simulink model "UG_Drive_System"  (R2019b)
settings: Solver=ode45  StartTime=0.0  StopTime=T_sim_d_ug  MaxStep=1e-5  RelTol=1e-3
values from neighbouring files (symbols this model uses):
  A_t = r * m * g * sin(theta)    [C2_Preliminary_Controller_Design.m]    (also in D1_Preliminary_Controller_Design.m; D2_Controller_Design.m; D3_PL_Controller_Design.m; D4_DPDZ_Controller_Design.m)
  B_t = r * C_r * m * g    [C2_Preliminary_Controller_Design.m]    (also in D1_Preliminary_Controller_Design.m = 0.0188352; D2_Controller_Design.m = 0.0188352; D3_PL_Controller_Design.m = 0.006309792; D4_DPDZ_Controller_Design.m = 0.006309792)
  C_t = r * 0.5 * rho_air * C_d * A    [C2_Preliminary_Controller_Design.m]    (also in D1_Preliminary_Controller_Design.m = 3.6e-05; D2_Controller_Design.m = 3.6e-05; D3_PL_Controller_Design.m = 3.6e-05; D4_DPDZ_Controller_Design.m = 3.6e-05)
  c_tv = r/((r.^2) * m + Jaxle)    [C2_Preliminary_Controller_Design.m]    (also in D1_Preliminary_Controller_Design.m; D2_Controller_Design.m; D3_PL_Controller_Design.m; D4_DPDZ_Controller_Design.m)
  delay_theta = 10    [D1_Preliminary_Controller_Design.m]    (also in D2_Controller_Design.m; D3_PL_Controller_Design.m; D4_DPDZ_Controller_Design.m)
  delay_v_x_ref = 1    [D1_Preliminary_Controller_Design.m]    (also in D2_Controller_Design.m; D3_PL_Controller_Design.m; D4_DPDZ_Controller_Design.m)
  eta_g_d = 1    [C2_Preliminary_Controller_Design.m]    (also in D1_Preliminary_Controller_Design.m = 0.95; D2_Controller_Design.m = 0.95; D3_PL_Controller_Design.m = 0.95; D4_DPDZ_Controller_Design.m = 0.95)
  i_a_max = 1.2    [D1_Preliminary_Controller_Design.m]    (also in D2_Controller_Design.m; D3_PL_Controller_Design.m; D4_DPDZ_Controller_Design.m)
  k_m_d =     [C2_Preliminary_Controller_Design.m]    (also in D1_Preliminary_Controller_Design.m = 0.02; D2_Controller_Design.m = 0.02; D3_PL_Controller_Design.m = 0.02; D4_DPDZ_Controller_Design.m = 0.02)
  L_a_d =     [C2_Preliminary_Controller_Design.m]    (also in D1_Preliminary_Controller_Design.m = 0.000278; D2_Controller_Design.m = 0.000278; D3_PL_Controller_Design.m = 0.000278; D4_DPDZ_Controller_Design.m = 0.000278)
  n_g_d =     [C2_Preliminary_Controller_Design.m]    (also in D1_Preliminary_Controller_Design.m = 50; D2_Controller_Design.m = 50; D3_PL_Controller_Design.m = 50; D4_DPDZ_Controller_Design.m = 50)
  pole_PL_d = exp(pole_PL_a * T_s)    [MPZ_PL.m]
  r =     [C2_Preliminary_Controller_Design.m]    (also in D1_Preliminary_Controller_Design.m = 0.06; D2_Controller_Design.m = 0.06; D3_PL_Controller_Design.m = 0.06; D4_DPDZ_Controller_Design.m = 0.06)
  R_a_d =     [C2_Preliminary_Controller_Design.m]    (also in D1_Preliminary_Controller_Design.m = 2.19; D2_Controller_Design.m = 2.19; D3_PL_Controller_Design.m = 2.19; D4_DPDZ_Controller_Design.m = 2.19)
  v_x_ref = 0.15    [D1_Preliminary_Controller_Design.m]    (also in D2_Controller_Design.m = 0.4; D3_PL_Controller_Design.m = 0.02; D4_DPDZ_Controller_Design.m = 0.02)
  zero_PL_d = exp(zero_PL_a * T_s)    [MPZ_PL.m]
undefined symbols (not defined in the file or in its folder): K_PL_d
settings Model: Creator=Conor  LastModifiedBy=Conor Healy
settings DataIOCC: SaveOutput=off  SignalLogging=off  DSMLogging=off  SaveTime=off  ReturnWorkspaceOutputs=off
settings SFSimCC: CustomCodeUndefinedFunction=UseInterfaceOnly

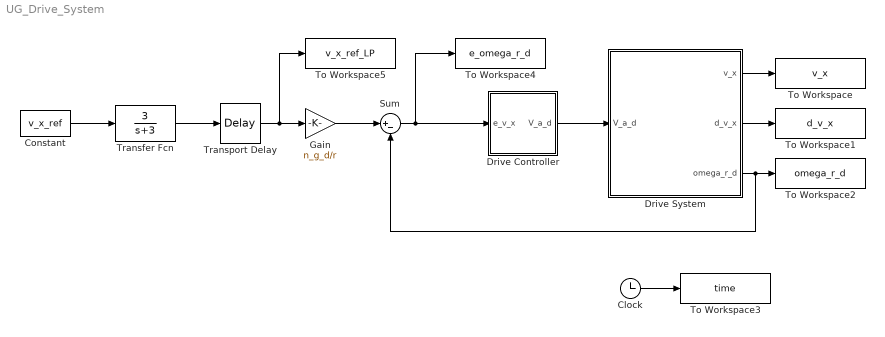
== system UG_Drive_System ==
  Clock : Clock
  Constant : Constant  Value=v_x_ref
  Drive Controller : Subsystem
  Drive System : Subsystem
  Gain : Gain  Gain=n_g_d/r
      settings: AttributesFormatString=%<Gain>
  Sum : Sum  Inputs=|+-
  To Workspace : ToWorkspace  VariableName=v_x  SampleTime=-1
  To Workspace1 : ToWorkspace  VariableName=d_v_x  SampleTime=-1
  To Workspace2 : ToWorkspace  VariableName=omega_r_d  SampleTime=-1
  To Workspace3 : ToWorkspace  VariableName=time  SampleTime=-1
  To Workspace4 : ToWorkspace  VariableName=e_omega_r_d  SampleTime=-1
  To Workspace5 : ToWorkspace  VariableName=v_x_ref_LP  SampleTime=-1
  Transfer Fcn : TransferFcn  Numerator=[3]  Denominator=[1 3]
  Transport Delay : TransportDelay  DelayTime=delay_v_x_ref  BufferSize=4096
  wires:
  Drive System/1(v_x) -> To Workspace/1
  Drive System/2(d_v_x) -> To Workspace1/1
  Drive System/3(omega_r_d) -> Sum/2, To Workspace2/1
  Gain/1 -> Sum/1
  Clock/1 -> To Workspace3/1
  Transport Delay/1 -> To Workspace5/1, Gain/1
  Sum/1 -> Drive Controller/1(e_v_x), To Workspace4/1
  Transfer Fcn/1 -> Transport Delay/1
  Constant/1 -> Transfer Fcn/1
  Drive Controller/1(V_a_d) -> Drive System/1(V_a_d)

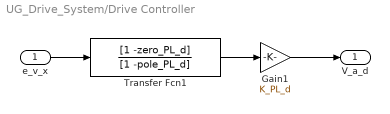
== system UG_Drive_System/Drive Controller ==
  e_v_x : Inport
  Gain1 : Gain  Gain=K_PL_d
      settings: AttributesFormatString=%<Gain>
  Transfer Fcn1 : TransferFcn  Numerator=[1 -zero_PL_d]  Denominator=[1 -pole_PL_d]
  V_a_d : Outport
  wires:
  Transfer Fcn1/1 -> Gain1/1
  Gain1/1 -> V_a_d/1
  e_v_x/1 -> Transfer Fcn1/1

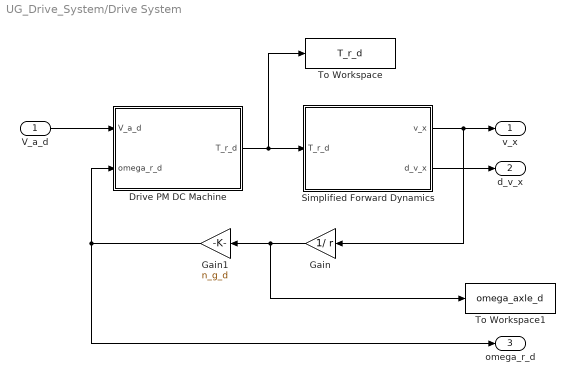
== system UG_Drive_System/Drive System ==
  V_a_d : Inport
  Drive PM DC Machine : Subsystem
  Gain : Gain  Gain=1/ r
      settings: AttributesFormatString=%<Gain>
  Gain1 : Gain  Gain=n_g_d
      settings: AttributesFormatString=%<Gain>
  Simplified Forward Dynamics : Subsystem
  To Workspace : ToWorkspace  VariableName=T_r_d  SampleTime=-1
  To Workspace1 : ToWorkspace  VariableName=omega_axle_d  SampleTime=-1
  v_x : Outport  VectorParamsAs1DForOutWhenUnconnected=off
  d_v_x : Outport  Port=2  VectorParamsAs1DForOutWhenUnconnected=off
  omega_r_d : Outport  Port=3  VectorParamsAs1DForOutWhenUnconnected=off
  wires:
  Drive PM DC Machine/1(T_r_d) -> To Workspace/1, Simplified Forward Dynamics/1(T_r_d)
  Simplified Forward Dynamics/1(v_x) -> Gain/1, v_x/1
  Simplified Forward Dynamics/2(d_v_x) -> d_v_x/1
  V_a_d/1 -> Drive PM DC Machine/1(V_a_d)
  Gain/1 -> To Workspace1/1, Gain1/1
  Gain1/1 -> omega_r_d/1, Drive PM DC Machine/2(omega_r_d)

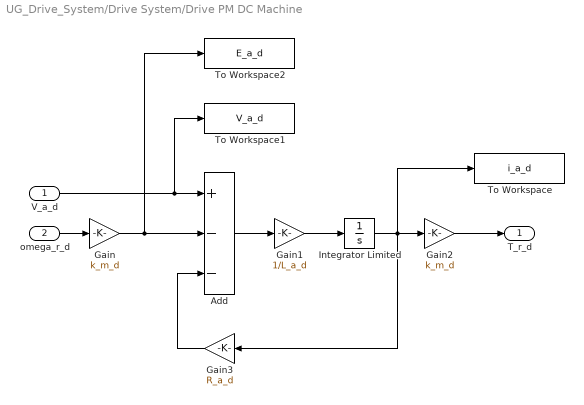
== system UG_Drive_System/Drive System/Drive PM DC Machine ==
  V_a_d : Inport
  omega_r_d : Inport  Port=2
  Add : Sum  Inputs=+--
  Gain : Gain  Gain=k_m_d
      settings: AttributesFormatString=%<Gain>
  Gain1 : Gain  Gain=1/L_a_d
      settings: AttributesFormatString=%<Gain>
  Gain2 : Gain  Gain=k_m_d
      settings: AttributesFormatString=%<Gain>
  Gain3 : Gain  Gain=R_a_d
      settings: AttributesFormatString=%<Gain>
  Integrator Limited : Integrator  LimitOutput=on  UpperSaturationLimit=i_a_max  LowerSaturationLimit=-i_a_max
  To Workspace : ToWorkspace  VariableName=i_a_d  SampleTime=-1
  To Workspace1 : ToWorkspace  VariableName=V_a_d  SampleTime=-1
  To Workspace2 : ToWorkspace  VariableName=E_a_d  SampleTime=-1
  T_r_d : Outport  VectorParamsAs1DForOutWhenUnconnected=off
  wires:
  V_a_d/1 -> To Workspace1/1, Add/1
  Gain/1 -> To Workspace2/1, Add/2
  omega_r_d/1 -> Gain/1
  Add/1 -> Gain1/1
  Gain1/1 -> Integrator Limited/1
  Integrator Limited/1 -> Gain2/1, To Workspace/1, Gain3/1
  Gain3/1 -> Add/3
  Gain2/1 -> T_r_d/1

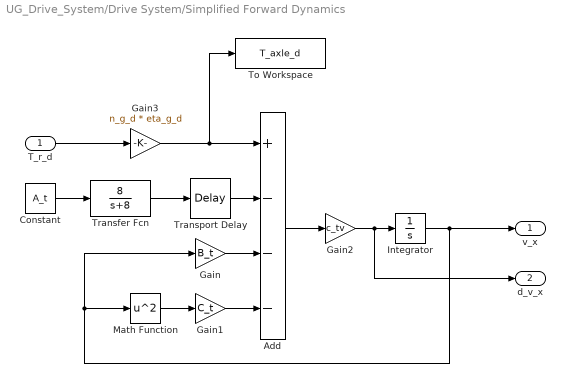
== system UG_Drive_System/Drive System/Simplified Forward Dynamics ==
  T_r_d : Inport
  Add : Sum  Inputs=+---
  Constant : Constant  Value=A_t
  Gain : Gain  Gain=B_t
  Gain1 : Gain  Gain=C_t
  Gain2 : Gain  Gain=c_tv
  Gain3 : Gain  Gain=n_g_d * eta_g_d
      settings: AttributesFormatString=%<Gain>
  Integrator : Integrator
  Math Function : Math  Operator=square  SaturateOnIntegerOverflow=on
  To Workspace : ToWorkspace  VariableName=T_axle_d  SampleTime=-1
  Transfer Fcn : TransferFcn  Numerator=[8]  Denominator=[1 8]
  Transport Delay : TransportDelay  DelayTime=delay_theta  BufferSize=4096
  v_x : Outport  VectorParamsAs1DForOutWhenUnconnected=off
  d_v_x : Outport  Port=2  VectorParamsAs1DForOutWhenUnconnected=off
  wires:
  Gain/1 -> Add/3
  Gain1/1 -> Add/4
  Gain3/1 -> To Workspace/1, Add/1
  T_r_d/1 -> Gain3/1
  Math Function/1 -> Gain1/1
  Add/1 -> Gain2/1
  Gain2/1 -> d_v_x/1, Integrator/1
  Integrator/1 -> v_x/1, Math Function/1, Gain/1
  Transport Delay/1 -> Add/2
  Constant/1 -> Transfer Fcn/1
  Transfer Fcn/1 -> Transport Delay/1
